simulink model "linear3DOF"  (R2025b)
settings: Solver=ode5  StartTime=0.0  StopTime=100  FixedStep=0.001  RelTol=1e-3
InitFcn:
  | % 定义车辆参数
  | m = 1370 + 89.9 + 65.2 + 22*4;       % 车辆质量 (kg)
  | % Vx = 120/3.6;        % 纵向速度 (m/s)
  | Cf = -4.487763550086564e+04 * 2;    % 前轴总侧偏刚度 (N/rad)
  | Cr = Cf;   % 后轴总侧偏刚度 (N/rad)
  | lf = 1.11;       % 质心到前轴距离 (m)
  | lr = 2.866-lf;       % 质心到后轴距离 (m)
  | Iz = 2315.3 + 0.08 + 0.08 + 0.8*4;      % 绕z轴转动惯量 (kg·m²)
  | Bf = 1.55;
  | Br = 1.55;
  | Re = 0.325;
undefined symbols (not defined in the file): speed_from_matlab
libraries: simulink_extras x2, Solver_SF x1, simulink x1
settings Model: Creator=23649  LastModifiedBy=23649

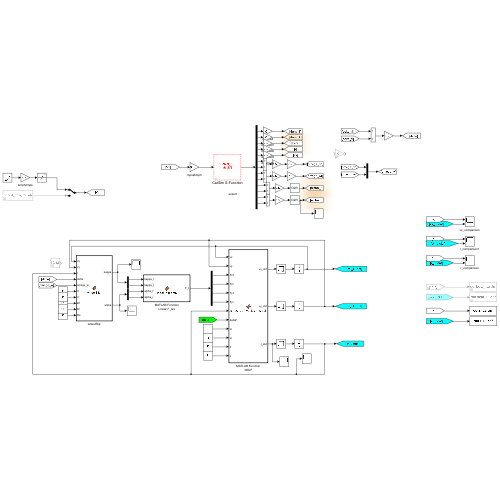
[thumbnail: Simulink's stored preview of the top-level diagram]
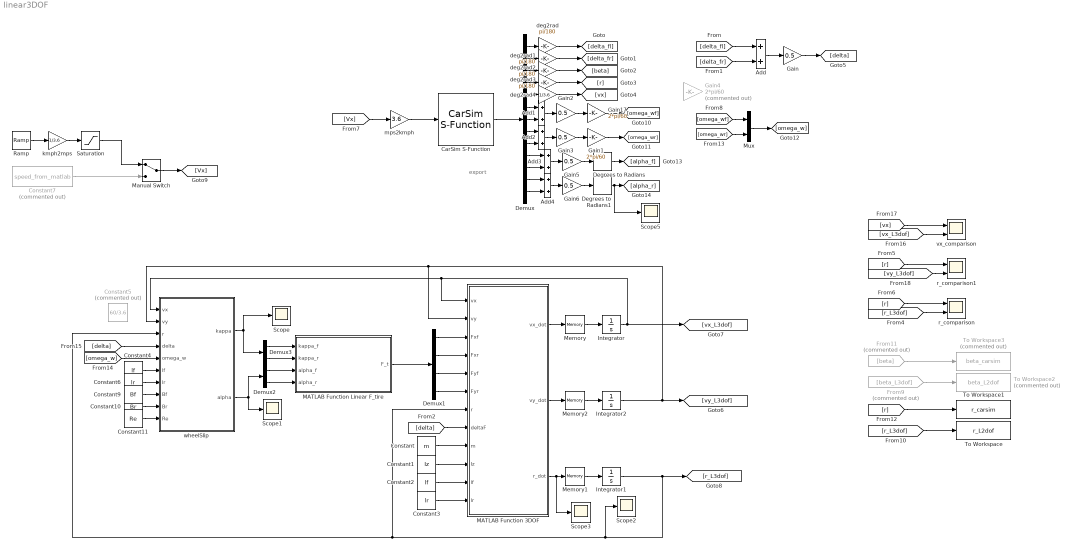
== system linear3DOF ==
  note: export
  Add{,1..4} (5 alike) : Sum
  CarSim S-Function : Solver_SF/CarSim S-Function  Priority=1  SIMFILE=simfile.sim  Run_RTs=off  vs_state_ind=Run  StopMode_ind=Vehicle Model
  Constant : Constant  Value=m
  Constant1 : Constant  Value=Iz
  Constant10 : Constant  Value=Br
  Constant11 : Constant  Value=Re
  Constant2 : Constant  Value=lf
  Constant3 : Constant  Value=lr
  Constant4 : Constant  Value=lf
  Constant5 : Constant  Commented=on  Value=60/3.6
  Constant6 : Constant  Value=lr
  Constant7 : Constant  Commented=on  Value=speed_from_matlab
  Constant9 : Constant  Value=Bf
  Degrees to Radians : simulink_extras/Transformations/Degrees to Radians
  Degrees to Radians1 : simulink_extras/Transformations/Degrees to Radians
  Demux : Demux  Outputs=13
  Demux1 : Demux
  Demux2 : Demux  Outputs=2
  Demux3 : Demux  Outputs=2
  From11 : From  Commented=on  GotoTag=beta
  From9 : From  Commented=on  GotoTag=beta_L3dof
  Gain{,2..3,5..6} (5 alike) : Gain  Gain=0.5
  Gain1 : Gain  Gain=2*pi/60
  Gain17 : Gain  Gain=2*pi/60
  Gain4 : Gain  Commented=on  Gain=2*pi/60
  Integrator : Integrator
  Integrator1 : Integrator
  Integrator2 : Integrator
  MATLAB Function 3DOF : MATLAB Function  TreatAsAtomicUnit=on
  MATLAB Function Linear F_tire : MATLAB Function  TreatAsAtomicUnit=on
  Manual Switch : ManualSwitch
  Memory : Memory
  Memory1 : Memory
  Memory2 : Memory
  Mux : Mux  Inputs=2
  Ramp : simulink/Sources/Ramp  slope=5  start=1  InitialOutput=0
  Saturation : Saturate  UpperLimit=20
  Scope{,1..3,5} (5 alike) : Scope
      Scope settings: ActiveDisplayYMinimum=-0.028952495123759275  ActiveDisplayYMaximum=0.011830288285428203  DataLoggingVariableName=ScopeData3
      Scope1 settings: ActiveDisplayYMinimum=-0.34571423576469579  ActiveDisplayYMaximum=0.42734599797227618  DataLoggingVariableName=ScopeData4
      Scope2 settings: ActiveDisplayYMinimum=-1  ActiveDisplayYMaximum=1  DataLoggingVariableName=ScopeData5
      Scope3 settings: ActiveDisplayYMinimum=-1  ActiveDisplayYMaximum=1  DataLoggingVariableName=ScopeData6
      Scope5 settings: ActiveDisplayYMinimum=-0.046490417382553315  ActiveDisplayYMaximum=0.049542184635143857  DataLoggingVariableName=ScopeData8
  To Workspace : ToWorkspace  VariableName=r_L2dof  SampleTime=-1
  To Workspace1 : ToWorkspace  VariableName=r_carsim  SampleTime=-1
  To Workspace2 : ToWorkspace  Commented=on  VariableName=beta_L2dof  SampleTime=-1
  To Workspace3 : ToWorkspace  Commented=on  VariableName=beta_carsim  SampleTime=-1
  deg2rad{,1..3} (4 alike) : Gain  Gain=pi/180
  deg2rad4 : Gain  Gain=1/3.6
  kmph2mps : Gain  Gain=1/3.6
  mps2kmph : Gain  Gain=3.6
  r_comparison : Scope  NumInputPorts=2
      settings: ActiveDisplayYMinimum=-0.45185424423810894  ActiveDisplayYMaximum=0.40684444921691254
  r_comparison1 : Scope  NumInputPorts=2
      settings: ActiveDisplayYMinimum=-0.23111502983023319  ActiveDisplayYMaximum=0.23036236303418919
  vx_comparison : Scope  NumInputPorts=2
      settings: ActiveDisplayYMinimum=-2.5675990368486441  ActiveDisplayYMaximum=22.926133567085074  DataLoggingVariableName=ScopeData2
  wheelSlip : MATLAB Function  TreatAsAtomicUnit=on
  wires:
  Constant2/1 -> MATLAB Function 3DOF/11(lf)
  Memory1/1 -> Integrator1/1
  Constant7/1 -> Manual Switch/2
  [r] -> r_comparison/1
  [delta_fr] -> Add/2
  [r] -> To Workspace1/1
  deg2rad3/1 -> [r]
  Add/1 -> Gain/1
  Memory/1 -> Integrator/1
  From11/1 -> To Workspace3/1
  [r_L3dof] -> r_comparison/2
  Demux/3 -> deg2rad2/1
  Integrator/1 -> MATLAB Function 3DOF/1(vx), wheelSlip/1(vx), [vx_L3dof]
  deg2rad/1 -> [delta_fl]
  Gain/1 -> [delta]
  deg2rad2/1 -> [beta]
  Constant3/1 -> MATLAB Function 3DOF/12(lr)
  [delta_fl] -> Add/1
  MATLAB Function 3DOF/1(vx_dot) -> Memory/1
  [Vx] -> mps2kmph/1
  mps2kmph/1 -> CarSim S-Function/1
  Demux/4 -> deg2rad3/1
  Manual Switch/1 -> [Vx]
  CarSim S-Function/1 -> Demux/1
  MATLAB Function 3DOF/3(r_dot) -> Scope3/1, Memory1/1
  Integrator1/1 -> [r_L3dof], Scope2/1, wheelSlip/3(r), MATLAB Function 3DOF/7(r)
  Constant1/1 -> MATLAB Function 3DOF/10(Iz)
  deg2rad1/1 -> [delta_fr]
  [r_L3dof] -> To Workspace/1
  Ramp/1 -> kmph2mps/1
  Demux/5 -> deg2rad4/1
  From9/1 -> To Workspace2/1
  Demux/1 -> deg2rad/1
  Demux/2 -> deg2rad1/1
  kmph2mps/1 -> Saturation/1
  Constant/1 -> MATLAB Function 3DOF/9(m)
  [delta] -> MATLAB Function 3DOF/8(deltaF)
  MATLAB Function 3DOF/2(vy_dot) -> Memory2/1
  Integrator2/1 -> MATLAB Function 3DOF/2(vy), wheelSlip/2(vy), [vy_L3dof]
  Memory2/1 -> Integrator2/1
  Demux1/4 -> MATLAB Function 3DOF/6(Fyr)
  Demux1/3 -> MATLAB Function 3DOF/5(Fyf)
  Demux1/2 -> MATLAB Function 3DOF/4(Fxr)
  Demux1/1 -> MATLAB Function 3DOF/3(Fxf)
  MATLAB Function Linear F_tire/1(F_t) -> Demux1/1
  wheelSlip/2(alpha) -> Demux2/1, Scope1/1
  wheelSlip/1(kappa) -> Demux3/1, Scope/1
  Constant4/1 -> wheelSlip/6(lf)
  Constant6/1 -> wheelSlip/7(lr)
  Constant10/1 -> wheelSlip/9(Br)
  Constant9/1 -> wheelSlip/8(Bf)
  Demux/8 -> Add2/1
  Demux/6 -> Add1/1
  Add1/1 -> Gain2/1
  Demux/7 -> Add1/2
  Demux/9 -> Add2/2
  Add2/1 -> Gain3/1
  Gain3/1 -> Gain1/1
  Gain2/1 -> Gain17/1
  Gain17/1 -> [omega_wf]
  Gain1/1 -> [omega_wr]
  [omega_wf] -> Mux/1
  [omega_wr] -> Mux/2
  Mux/1 -> [omega_w]
  [omega_w] -> wheelSlip/5(omega_w)
  [delta] -> wheelSlip/4(delta)
  Constant11/1 -> wheelSlip/10(Re)
  [vy_L3dof] -> r_comparison1/2
  [r] -> r_comparison1/1
  [vx] -> vx_comparison/1
  [vx_L3dof] -> vx_comparison/2
  Demux3/2 -> MATLAB Function Linear F_tire/2(kappa_r)
  Demux3/1 -> MATLAB Function Linear F_tire/1(kappa_f)
  Saturation/1 -> Manual Switch/1
  deg2rad4/1 -> [vx]
  Add4/1 -> Gain6/1
  Demux/11 -> Add3/2
  Demux/10 -> Add3/1
  Demux/12 -> Add4/1
  Demux/13 -> Add4/2
  Add3/1 -> Gain5/1
  Gain5/1 -> Degrees to Radians/1
  Gain6/1 -> Degrees to Radians1/1
  Degrees to Radians/1 -> [alpha_f]
  Degrees to Radians1/1 -> Scope5/1, [alpha_r]
  Demux2/2 -> MATLAB Function Linear F_tire/4(alpha_r)
  Demux2/1 -> MATLAB Function Linear F_tire/3(alpha_f)

== matlab function linear3DOF/MATLAB Function Linear F_tire ==
  data: kappa_f input; F_t output; kappa_r input; alpha_f input; alpha_r input
function F_t = linearTrieForce(kappa_f, kappa_r, alpha_f, alpha_r)
    
    % 轮胎刚度参数
    Cxf =  37500*2;
    Cyf = -90000 * 2;
    
    Cxr = Cxf;
    Cyr = Cyf;

    % kappa_f = (Re * omega_tf - v_xtf) / abs(v_xtf);
    % kappa_r = (Re * omega_tr - v_xtr) / abs(v_xtr);
    % 
    % alpha_f = atan(-(vx * sin(deltaF) - vy * cos(deltaF)) / (vx * cos(deltaF) + vy * sin(deltaF)));
    % alpha_r = atan(-(vx * sin(deltaR) - vy * cos(deltaR)) / (vx * cos(deltaR) + vy * sin(deltaR)));

    % 前轮纵侧向力
    Fxf = Cxf * kappa_f;
    Fyf = Cyf * alpha_f;
    
    % 后轮纵侧向力
    Fxr = Cxr * kappa_r;
    Fyr = Cyr * alpha_r;
    

    % 轮胎力限制
    [Fxf, Fyf] = limitedTireForce(Fxf, Fyf);
    [Fxr, Fyr] = limitedTireForce(Fxr, Fyr);


    % 轮胎力 前纵，后纵，前侧，后侧
    F_t = [Fxf, Fxr, Fyf, Fyr];
end 

function [Fx, Fy] = limitedTireForce(Fx, Fy)

    Fmax =  1500 * 9.8/2;

    if (Fx^2 + Fy^2) > Fmax^2
        wx = Fx/sqrt(Fx^2 + Fy^2);
        wy = Fy/sqrt(Fx^2 + Fy^2);
        Fx = wx*Fmax;
        Fy = wy*Fmax;
    end

end

== matlab function linear3DOF/MATLAB Function 3DOF ==
  data: vx input; vy input; Fxf input; Fxr input; Fyf input; Fyr input; r input; deltaF input; vx_dot output; vy_dot output; r_dot output; m input; Iz input; lf input; lr input
function [vx_dot, vy_dot, r_dot] = three_dof_vehicle_model(vx, vy, Fxf, Fxr, Fyf, Fyr, r, deltaF, m, Iz, lf, lr)
    % 线性二自由度车辆动力学模型
    % 输入：
    %   β: 质心侧偏角 (rad)
    %   r: 横摆角速度 (rad/s)
    %   delta：前轮转角 (rad)
    %   Vx: 纵向速度 (m/s)
    %   整车params - 参数结构体，包含：
    %       m: 车辆质量 (kg)
    %       Iz: 绕z轴转动惯量 (kg·m²)
    %       lf: 质心到前轴距离 (m)
    %       lr: 质心到后轴距离 (m)
    %       Cf: 前轴总侧偏刚度 (N/rad)
    %       Cr: 后轴总侧偏刚度 (N/rad)
    % 输出：
    %   beta_dot, r_dot - 状态导数 [dβ/dt; dr/dt]
  
    
    % 空气阻力
    A = 2.2;
    D = 1.206;
    CFx = 0.3;
    % CFy = 2;
    Q = D * vx * abs(vx) / 2;
    Fx_aero = - CFx * A * Q; 

    % 计算状态导数

    vx_dot =  vy*r + (Fxf * cos(deltaF) - Fyf * sin(deltaF) + Fxr + Fx_aero) / m;

    vy_dot = -vx*r + (Fxf * sin(deltaF) + Fyf * cos(deltaF) + Fyr) / m;

    r_dot = (lf*(Fxf * sin(deltaF) + Fyf * cos(deltaF)) - lr * Fyr) / Iz;

end

== matlab function linear3DOF/wheelSlip ==
  data: kappa output; vx input; vy input; r input; delta input; omega_w input; lf input; lr input; Bf input; Br input; alpha output; Re input
function [kappa, alpha] = wheelSlip(vx, vy, r, delta, omega_w, lf, lr, Bf, Br, Re)
    

    
    model = 2;                          %前后两个车轮
    if model == 2
        B = [0; 0];
        l = [lf; -lr];
        if isscalar(delta)
            delta = [delta; 0];
        end
    elseif  model == 4                  %前后左右四个车轮
        B = [-Bf;Bf;-Br;Br]/2;
        l = [lf;lf;-lr;-lr];
        if length(delta) == 2
            delta = [delta(1); delta(2); 0; 0];
        end
    end

    vwx_V = vx - B*r;
    vwy_V = vy + l*r;
    
    vwx_W =  vwx_V .* cos(delta) + vwy_V .* sin(delta);
    vwy_W = -vwx_V .* sin(delta) + vwy_V .* cos(delta);

    vwx_W(abs(vwx_W)<0.001) = 0.001;
    alpha = atan(vwy_W ./ vwx_W);

    % vwx_V(vwx_V(:,1) == 0) = 1e-3;
    % alpha = atan(vwy_V ./ vwx_V) - delta;

    kappa = (Re*omega_w - vwx_W) ./ abs(vwx_W);
    
end
